simulink model "m2fsm_2_rust"  (R2022b)
settings: Solver=FixedStepDiscrete  StartTime=0.0  StopTime=5  FixedStep=deltaT  RelTol=1e-3
undefined symbols (not defined in the file or in its folder): A_oa_pec, A_oa_pzt, A_S7_pzt, B_oa_pec, B_oa_pzt, B_S7_pzt, C_oa_pec, C_oa_pzt, C_S7_pzt, D_oa_pec, D_oa_pzt, D_S7_pzt, fc, k2p_stiff, Km2pS1_dec, m2p_Cfb_d, to_diff_m2p_F, Ts, tt7
settings Model: SimulationMode=accelerator  Creator=RRomano  LastModifiedBy=rromano
settings DataIOCC: SaveOutput=off  SignalLogging=off  DSMLogging=off  SaveTime=off  ReturnWorkspaceOutputs=off
settings OptimizationCC: DefaultParameterBehavior=Inlined  GainParamInheritBuiltInType=on  UseFloatMulNetSlope=on  UseSpecifiedMinMax=on  InlineInvariantSignals=on  StrengthReduction=on  PassReuseOutputArgsAs=Individual arguments  ZeroExternalMemoryAtStartup=off  ZeroInternalMemoryAtStartup=off  NoFixptDivByZeroProtection=on  EfficientFloat2IntCast=on  LifeSpan=1000  SimCompilerOptimization=on  AccelVerboseBuild=on  OptimizeBlockOrder=speed  OptimizationPriority=Speed  OptimizationCustomize=off  MultiThreadedLoops=on  EfficientTunableParamExpr=on
settings DebuggingCC: InheritedTsInSrcMsg=none  MultiTaskRateTransMsg=warning  ParameterTunabilityLossMsg=error  UnconnectedInputMsg=warning  UnconnectedOutputMsg=warning  UnconnectedLineMsg=warning  SFUnexpectedBacktrackingDiag=warning  SFNoUnconditionalDefaultTransitionDiag=warning  SFExecutionAtInitializationDiag=none  SFMachineParentedDataDiag=warning  ArithmeticOperatorsInVariantConditions=warning
settings HardwareCC: ProdBitPerLong=64  ProdLongLongMode=on  ProdHWDeviceType=Intel->x86-64 (Linux 64)  TargetBitPerLong=64  TargetBitPerPointer=64  TargetBitPerSizeT=64  TargetBitPerPtrDiffT=64  TargetLongLongMode=on  TargetIntDivRoundTo=Zero  TargetEndianess=LittleEndian  TargetWordSize=64  TargetHWDeviceType=MATLAB Host  ProdEqTarget=off
settings ModelReferenceCC: EnableRefExpFcnMdlSchedulingChecks=on
settings SFSimCC: MATLABDynamicMemAlloc=off  CustomCodeUndefinedFunction=UseInterfaceOnly
settings RTWCC: Description=Embedded Coder  SystemTargetFile=ert.tlc  GenCodeOnly=on  GenerateMakefile=off  TemplateMakefile=ert_default_tmf  GenerateReport=on  BuildConfiguration=Faster Runs  RTWCompilerOptimization=on  CheckMdlBeforeBuild=Warning
settings CodeAppCC: ForceParamTrailComments=on  IgnoreCustomStorageClasses=off  OperatorAnnotations=on  SimulinkDataObjDesc=on  SFDataObjDesc=on  InsertBlockDesc=on
settings ERTTargetCC: TargetLangStandard=C99 (ISO)  GenerateSampleERTMain=on  CombineSignalStateStructs=on  SuppressErrorStatus=on  CodeInterfacePackaging=Reusable function  SupportNonFinite=off  SupportComplex=off  InlinedParameterPlacement=NonHierarchical  RootIOFormat=Structure reference  ERTCustomFileTemplate=example_file_process.tlc

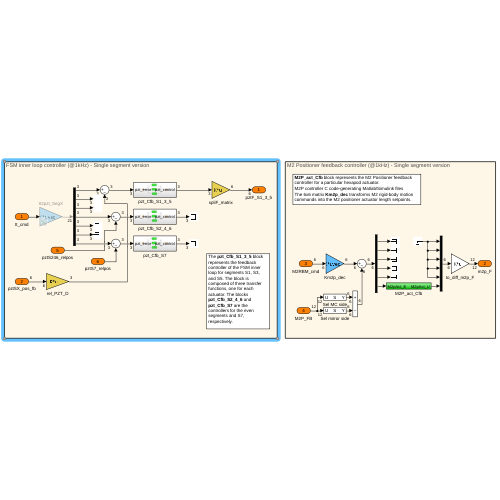
[thumbnail: Simulink's stored preview of the top-level diagram]
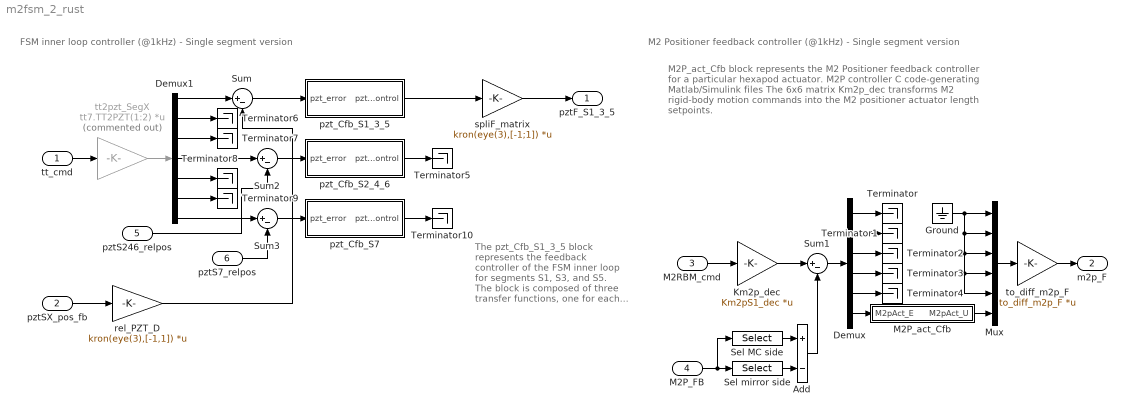
== system m2fsm_2_rust ==
  note: The pzt_Cfb_S1_3_5 block represents the feedback controller of the FSM inner loop for segments S1, S3, and S5. The block is composed of three transfer functions, one for each actuator. The blocks pzt_Cfb_S2_4_6 and pzt_Cfb_S7 are the controllers for the even segments and S7, respectively.
  note: FSM inner loop controller (@1kHz) - Single segment version
  note: M2 Positioner feedback controller (@1kHz) - Single segment version
  note: M2P_act_Cfb block represents the M2 Positioner feedback controller for a particular hexapod actuator.
      | M2P controller C code-generating Matlab/Simulink files
      | The 6x6 matrix Km2p_dec transforms M2 rigid-body motion commands into the M2 positioner actuator length setpoints.
  tt_cmd : Inport
  pztSX_pos_fb : Inport  Port=2  PortDimensions=3*2
  M2RBM_cmd : Inport  Port=3  Interpolate=off
  M2P_FB : Inport  Port=4
  pztS246_relpos : Inport  Port=5
  pztS7_relpos : Inport  Port=6
  Add : Sum  Inputs=+-
  Demux : Demux  Outputs=6
  Demux1 : Demux  Outputs=3*ones(1,7)
  Ground : Ground
  Km2p_dec : Gain  Gain=Km2pS1_dec  Multiplication=Matrix(K*u) (u vector)
  M2P_act_Cfb : Subsystem
  Mux : Mux  Inputs=6
  Sel MC side : Selector  InputPortWidth=12  IndexOptions=Index vector (dialog)  Indices=[1:2:12]  OutputSizes=1
  Sel mirror side : Selector  InputPortWidth=12  IndexOptions=Index vector (dialog)  Indices=[2:2:12]  OutputSizes=1
  Sum{,1..3} (4 alike) : Sum  Inputs=|+-
  Terminator{,1..10} (11 alike) : Terminator
  pzt_Cfb_S1_3_5 : Subsystem
  pzt_Cfb_S2_4_6 : Subsystem
  pzt_Cfb_S7 : Subsystem
  rel_PZT_D : Gain  Gain=kron(eye(3),[-1,1])  Multiplication=Matrix(K*u)
  spliF_matrix : Gain  Gain=kron(eye(3),[-1;1])  Multiplication=Matrix(K*u)
  to_diff_m2p_F : Gain  Gain=to_diff_m2p_F  Multiplication=Matrix(K*u)
  tt2pzt_SegX : Gain  Commented=on  Gain=tt7.TT2PZT(1:2)  Multiplication=Matrix(K*u) (u vector)
  pztF_S1_3_5 : Outport  VectorParamsAs1DForOutWhenUnconnected=off
  m2p_F : Outport  Port=2  VectorParamsAs1DForOutWhenUnconnected=off
  wires:
  M2RBM_cmd/1 -> Km2p_dec/1
  Km2p_dec/1 -> Sum1/1
  Add/1 -> Sum1/2
  Sum1/1 -> Demux/1
  Mux/1 -> to_diff_m2p_F/1
  to_diff_m2p_F/1 -> m2p_F/1
  Sel MC side/1 -> Add/1
  Sel mirror side/1 -> Add/2
  M2P_FB/1 -> Sel MC side/1, Sel mirror side/1
  Demux/1 -> Terminator/1
  Demux/2 -> Terminator1/1
  Demux/3 -> Terminator2/1
  Demux/4 -> Terminator3/1
  Demux/5 -> Terminator4/1
  Ground/1 -> Mux/5, Mux/4, Mux/3, Mux/2, Mux/1
  Demux/6 -> M2P_act_Cfb/1(M2pAct_E)
  M2P_act_Cfb/1(M2pAct_U) -> Mux/6
  spliF_matrix/1 -> pztF_S1_3_5/1
  tt_cmd/1 -> tt2pzt_SegX/1
  rel_PZT_D/1 -> Sum/2
  pztSX_pos_fb/1 -> rel_PZT_D/1
  Demux1/2 -> Terminator6/1
  Demux1/3 -> Terminator7/1
  Demux1/5 -> Terminator8/1
  Demux1/6 -> Terminator9/1
  Demux1/1 -> Sum/1
  tt2pzt_SegX/1 -> Demux1/1
  Sum/1 -> pzt_Cfb_S1_3_5/1(pzt_error)
  Sum2/1 -> pzt_Cfb_S2_4_6/1(pzt_error)
  Demux1/4 -> Sum2/1
  Sum3/1 -> pzt_Cfb_S7/1(pzt_error)
  Demux1/7 -> Sum3/1
  pztS7_relpos/1 -> Sum3/2
  pztS246_relpos/1 -> Sum2/2
  pzt_Cfb_S1_3_5/1(pzt_control) -> spliF_matrix/1
  pzt_Cfb_S7/1(pzt_control) -> Terminator10/1
  pzt_Cfb_S2_4_6/1(pzt_control) -> Terminator5/1

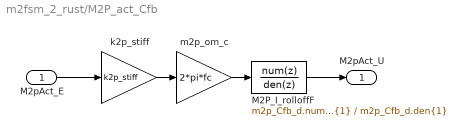
== system m2fsm_2_rust/M2P_act_Cfb ==
  M2pAct_E : Inport
  M2P_I_rolloffF : DiscreteTransferFcn  Numerator=m2p_Cfb_d.num{1}  Denominator=m2p_Cfb_d.den{1}  SampleTime=m2p_Cfb_d.Ts
  k2p_stiff : Gain  Gain=k2p_stiff
  m2p_om_c : Gain  Gain=2*pi*fc
  M2pAct_U : Outport
  wires:
  M2P_I_rolloffF/1 -> M2pAct_U/1
  M2pAct_E/1 -> k2p_stiff/1
  k2p_stiff/1 -> m2p_om_c/1
  m2p_om_c/1 -> M2P_I_rolloffF/1

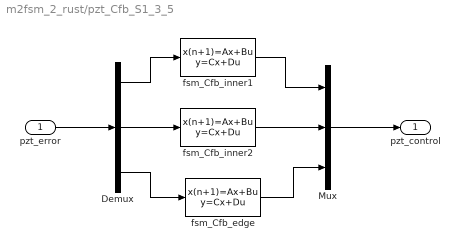
== system m2fsm_2_rust/pzt_Cfb_S1_3_5 ==
  pzt_error : Inport
  Demux : Demux  Outputs=3
  Mux : Mux  Inputs=3
  fsm_Cfb_edge : DiscreteStateSpace  A=A_oa_pec  B=B_oa_pec  C=C_oa_pec  D=D_oa_pec  SampleTime=Ts
  fsm_Cfb_inner1 : DiscreteStateSpace  A=A_oa_pzt  B=B_oa_pzt  C=C_oa_pzt  D=D_oa_pzt  SampleTime=Ts
  fsm_Cfb_inner2 : DiscreteStateSpace  A=A_oa_pzt  B=B_oa_pzt  C=C_oa_pzt  D=D_oa_pzt  SampleTime=Ts
  pzt_control : Outport  VectorParamsAs1DForOutWhenUnconnected=off
  wires:
  fsm_Cfb_inner1/1 -> Mux/1
  fsm_Cfb_edge/1 -> Mux/3
  Demux/1 -> fsm_Cfb_inner1/1
  Demux/3 -> fsm_Cfb_edge/1
  Demux/2 -> fsm_Cfb_inner2/1
  fsm_Cfb_inner2/1 -> Mux/2
  pzt_error/1 -> Demux/1
  Mux/1 -> pzt_control/1

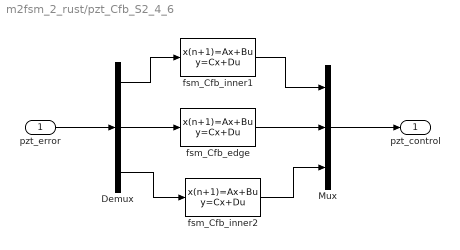
== system m2fsm_2_rust/pzt_Cfb_S2_4_6 ==
  pzt_error : Inport
  Demux : Demux  Outputs=3
  Mux : Mux  Inputs=3
  fsm_Cfb_edge : DiscreteStateSpace  A=A_oa_pec  B=B_oa_pec  C=C_oa_pec  D=D_oa_pec  SampleTime=Ts
  fsm_Cfb_inner1 : DiscreteStateSpace  A=A_oa_pzt  B=B_oa_pzt  C=C_oa_pzt  D=D_oa_pzt  SampleTime=Ts
  fsm_Cfb_inner2 : DiscreteStateSpace  A=A_oa_pzt  B=B_oa_pzt  C=C_oa_pzt  D=D_oa_pzt  SampleTime=Ts
  pzt_control : Outport  VectorParamsAs1DForOutWhenUnconnected=off
  wires:
  fsm_Cfb_inner1/1 -> Mux/1
  Demux/1 -> fsm_Cfb_inner1/1
  Demux/2 -> fsm_Cfb_edge/1
  fsm_Cfb_edge/1 -> Mux/2
  pzt_error/1 -> Demux/1
  Mux/1 -> pzt_control/1
  fsm_Cfb_inner2/1 -> Mux/3
  Demux/3 -> fsm_Cfb_inner2/1

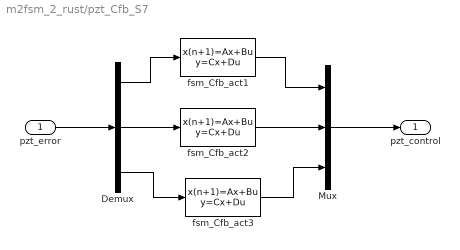
== system m2fsm_2_rust/pzt_Cfb_S7 ==
  pzt_error : Inport
  Demux : Demux  Outputs=3
  Mux : Mux  Inputs=3
  fsm_Cfb_act1 : DiscreteStateSpace  A=A_S7_pzt  B=B_S7_pzt  C=C_S7_pzt  D=D_S7_pzt  SampleTime=Ts
  fsm_Cfb_act2 : DiscreteStateSpace  A=A_S7_pzt  B=B_S7_pzt  C=C_S7_pzt  D=D_S7_pzt  SampleTime=Ts
  fsm_Cfb_act3 : DiscreteStateSpace  A=A_S7_pzt  B=B_S7_pzt  C=C_S7_pzt  D=D_S7_pzt  SampleTime=Ts
  pzt_control : Outport  VectorParamsAs1DForOutWhenUnconnected=off
  wires:
  fsm_Cfb_act1/1 -> Mux/1
  Demux/1 -> fsm_Cfb_act1/1
  Demux/2 -> fsm_Cfb_act2/1
  fsm_Cfb_act2/1 -> Mux/2
  pzt_error/1 -> Demux/1
  Mux/1 -> pzt_control/1
  fsm_Cfb_act3/1 -> Mux/3
  Demux/3 -> fsm_Cfb_act3/1
